simulink model "EsquemaFeedforward"  (R2017a)
settings: Solver=VariableStepAuto  StartTime=0.0  StopTime=50  RelTol=1e-3
settings Model: Creator=julia  LastModifiedBy=julia

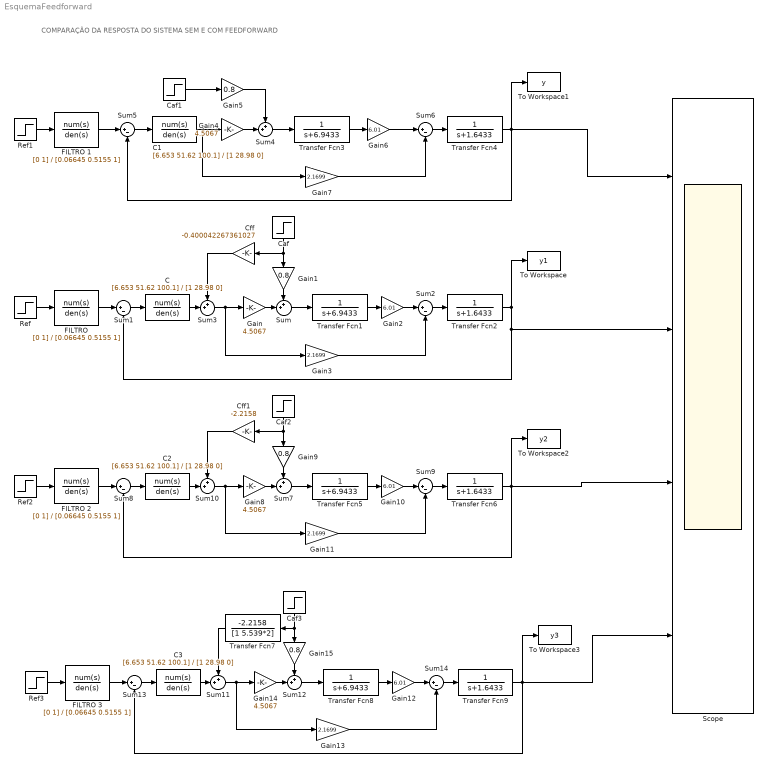
== system EsquemaFeedforward ==
  note: COMPARAÇÃO DA RESPOSTA DO SISTEMA SEM E COM FEEDFORWARD
  C{,1..3} (4 alike) : TransferFcn  Numerator=[6.653 51.62 100.1]  Denominator=[1 28.98 0]
  Caf{,1..3} (4 alike) : Step  Time=20  SampleTime=0
  Cff : Gain  Gain=-0.400042267361027
  Cff1 : Gain  Gain=-2.2158
  FILTRO {,1..3} (4 alike) : TransferFcn  Numerator=[0 1]  Denominator=[0.06645 0.5155 1]
  Gain{,4,8,14} (4 alike) : Gain  Gain=4.5067
  Gain{1,5,9,15} (4 alike) : Gain  Gain=0.8
  Gain{2,6,10,12} (4 alike) : Gain  Gain=6.01
  Gain{3,7,11,13} (4 alike) : Gain  Gain=2.1699
  Ref{,1..3} (4 alike) : Step  Time=0  SampleTime=0
  Scope : Scope  NumInputPorts=4
  Sum{,3..4,7,10..12} (7 alike) : Sum  Inputs=++|
  Sum{1..2,5..6,8..9,13..14} (8 alike) : Sum  Inputs=|+-
  To Workspace : ToWorkspace  VariableName=y1  SaveFormat=Timeseries  SampleTime=-1
  To Workspace1 : ToWorkspace  VariableName=y  SaveFormat=Timeseries  SampleTime=-1
  To Workspace2 : ToWorkspace  VariableName=y2  SaveFormat=Timeseries  SampleTime=-1
  To Workspace3 : ToWorkspace  VariableName=y3  SaveFormat=Timeseries  SampleTime=-1
  Transfer Fcn{1,3,5,8} (4 alike) : TransferFcn  Denominator=[1 6.9433]
  Transfer Fcn{2,4,6,9} (4 alike) : TransferFcn  Denominator=[1 1.6433]
  Transfer Fcn7 : TransferFcn  Numerator=[0 -2.2158]  Denominator=[1 5.539*2]
  wires:
  Transfer Fcn2/1 -> Sum1/2, Scope/2, To Workspace/1
  Gain3/1 -> Sum2/2
  Gain/1 -> Sum/2
  Transfer Fcn1/1 -> Gain2/1
  "FILTRO "/1 -> Sum1/1
  Caf/1 -> Gain1/1, Cff/1
  Gain2/1 -> Sum2/1
  Gain1/1 -> Sum/1
  Sum/1 -> Transfer Fcn1/1
  Ref/1 -> "FILTRO "/1
  Sum1/1 -> C/1
  Sum2/1 -> Transfer Fcn2/1
  C/1 -> Sum3/2
  Cff/1 -> Sum3/1
  Sum3/1 -> Gain3/1, Gain/1
  Transfer Fcn4/1 -> Scope/1, To Workspace1/1, Sum5/2
  Gain7/1 -> Sum6/2
  Gain4/1 -> Sum4/2
  Transfer Fcn3/1 -> Gain6/1
  FILTRO 1/1 -> Sum5/1
  Caf1/1 -> Gain5/1
  Gain6/1 -> Sum6/1
  C1/1 -> Gain7/1, Gain4/1
  Gain5/1 -> Sum4/1
  Sum4/1 -> Transfer Fcn3/1
  Ref1/1 -> FILTRO 1/1
  Sum5/1 -> C1/1
  Sum6/1 -> Transfer Fcn4/1
  Sum10/1 -> Gain8/1, Gain11/1
  Cff1/1 -> Sum10/1
  C2/1 -> Sum10/2
  Sum9/1 -> Transfer Fcn6/1
  Sum8/1 -> C2/1
  Ref2/1 -> FILTRO 2/1
  Sum7/1 -> Transfer Fcn5/1
  Gain9/1 -> Sum7/1
  Gain10/1 -> Sum9/1
  Caf2/1 -> Cff1/1, Gain9/1
  FILTRO 2/1 -> Sum8/1
  Transfer Fcn5/1 -> Gain10/1
  Gain8/1 -> Sum7/2
  Gain11/1 -> Sum9/2
  Transfer Fcn6/1 -> Scope/3, Sum8/2, To Workspace2/1
  Transfer Fcn9/1 -> Scope/4, To Workspace3/1, Sum13/2
  Gain13/1 -> Sum14/2
  Gain14/1 -> Sum12/2
  Transfer Fcn8/1 -> Gain12/1
  FILTRO 3/1 -> Sum13/1
  Caf3/1 -> Transfer Fcn7/1, Gain15/1
  Gain12/1 -> Sum14/1
  Gain15/1 -> Sum12/1
  Sum12/1 -> Transfer Fcn8/1
  Ref3/1 -> FILTRO 3/1
  Sum13/1 -> C3/1
  Sum14/1 -> Transfer Fcn9/1
  C3/1 -> Sum11/2
  Transfer Fcn7/1 -> Sum11/1
  Sum11/1 -> Gain13/1, Gain14/1
